simulink model "dynsim_edo_drag_gravity"  (R2020a)
settings: Solver=FixedStepAuto  StartTime=0.0  StopTime=10.0  FixedStep=0.001  RelTol=1e-3
libraries: robotlib x12, robotmaniplib x3
settings Model: Creator=bascetta  LastModifiedBy=alberto
settings OptimizationCC: EnhancedBackFolding=on  PassReuseOutputArgsAs=Individual arguments  ZeroExternalMemoryAtStartup=off  ZeroInternalMemoryAtStartup=off  MaxStackSize=64  OptimizeBlockOrder=speed  DifferentSizesBufferReuse=on  OptimizationCustomize=off  EfficientTunableParamExpr=on
settings DebuggingCC: ParameterTunabilityLossMsg=error
settings HardwareCC: ProdBitPerPointer=32  ProdBitPerSizeT=32  ProdBitPerPtrDiffT=32  ProdLargestAtomicFloat=None  ProdIntDivRoundTo=Undefined  ProdEndianess=Unspecified  ProdWordSize=32  ProdHWDeviceType=Generic->Unspecified (assume 32-bit Generic)
settings RTWCC: SystemTargetFile=ert.tlc  HardwareBoard=Robot Operating System (ROS)  TemplateMakefile=ert_default_tmf  GenerateReport=on  Toolchain=Catkin  IncludeHyperlinkInReport=on  LaunchReport=on  TargetLang=C++  GenerateTraceInfo=on  GenerateTraceReport=on  GenerateTraceReportSl=on  GenerateTraceReportSf=on  GenerateTraceReportEml=on
settings CodeAppCC: ForceParamTrailComments=on  IgnoreCustomStorageClasses=off  OperatorAnnotations=on  SimulinkDataObjDesc=on  SFDataObjDesc=on  InsertBlockDesc=on
settings ERTTargetCC: SupportContinuousTime=on  SupportVariableSizeSignals=on

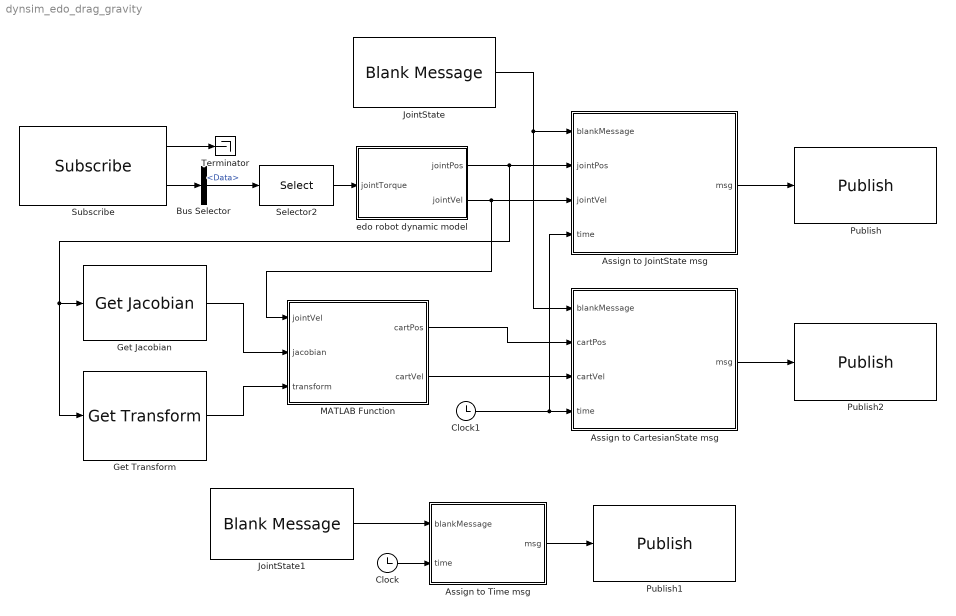
== system dynsim_edo_drag_gravity ==
  Assign to CartesianState msg : MATLAB Function  TreatAsAtomicUnit=on
  Assign to JointState msg : MATLAB Function  TreatAsAtomicUnit=on
  Assign to Time msg : MATLAB Function  TreatAsAtomicUnit=on
  Bus Selector : BusSelector  OutputSignals=Data
  Clock : Clock
  Clock1 : Clock
  Get Jacobian : robotmaniplib/Get Jacobian  RigidBodyTree=robot_edo  EndEffector=link_4  SimulateUsing=Interpreted execution
      settings: SourceProductBaseCode=RO
  Get Transform : robotmaniplib/Get Transform  RigidBodyTree=robot_edo  SourceBody=link_4  TargetBody=base_link  SimulateUsing=Interpreted execution
  JointState : robotlib/Blank Message  messageClass=Message  entityType=sensor_msgs/JointState  messageType=sensor_msgs/JointState  SampleTime=inf
  JointState1 : robotlib/Blank Message  messageClass=Message  entityType=rosgraph_msgs/Clock  messageType=rosgraph_msgs/Clock  SampleTime=inf
  MATLAB Function : MATLAB Function  TreatAsAtomicUnit=on
  Publish : robotlib/Publish  topicSource=Specify your own  topic=/joint_states  messageType=sensor_msgs/JointState  messageQueueLength=1
  Publish1 : robotlib/Publish  topicSource=Specify your own  topic=/clock  messageType=rosgraph_msgs/Clock  messageQueueLength=1
  Publish2 : robotlib/Publish  topicSource=Specify your own  topic=/cartesian_states  messageType=sensor_msgs/JointState  messageQueueLength=1
  Selector2 : Selector  IndexOptions=Starting index (dialog)  Indices=[2]  OutputSizes=3
  Subscribe : robotlib/Subscribe  topicSource=Specify your own  topic=/joint_torque  messageType=std_msgs/Float64MultiArray  sampleTime=-1  messageQueueLength=1
  Terminator : Terminator
  edo robot dynamic model : Subsystem
  wires:
  JointState1/1 -> Assign to Time msg/1(blankMessage)
  Assign to Time msg/1(msg) -> Publish1/1
  Subscribe/2 -> Bus Selector/1
  Subscribe/1 -> Terminator/1
  Selector2/1 -> edo robot dynamic model/1(jointTorque)
  Assign to JointState msg/1(msg) -> Publish/1
  edo robot dynamic model/2(jointVel) -> MATLAB Function/1(jointVel), Assign to JointState msg/3(jointVel)
  Bus Selector/1 -> Selector2/1  "<Data>"
  edo robot dynamic model/1(jointPos) -> Get Transform/1, Get Jacobian/1, Assign to JointState msg/2(jointPos)
  Clock/1 -> Assign to Time msg/2(time)
  Clock1/1 -> Assign to CartesianState msg/4(time), Assign to JointState msg/4(time)
  MATLAB Function/2(cartVel) -> Assign to CartesianState msg/3(cartVel)
  Assign to CartesianState msg/1(msg) -> Publish2/1
  MATLAB Function/1(cartPos) -> Assign to CartesianState msg/2(cartPos)
  JointState/1 -> Assign to CartesianState msg/1(blankMessage), Assign to JointState msg/1(blankMessage)
  Get Jacobian/1 -> MATLAB Function/2(jacobian)
  Get Transform/1 -> MATLAB Function/3(transform)

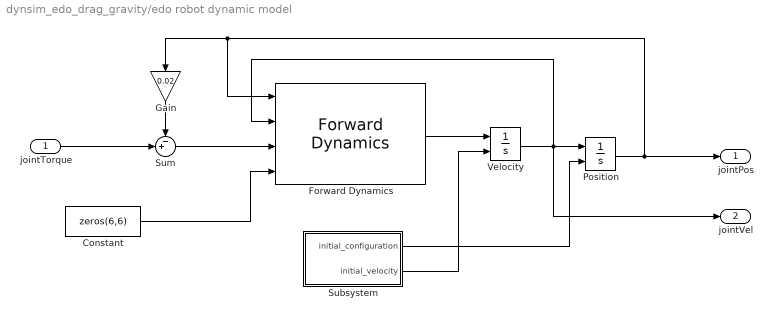
== system dynsim_edo_drag_gravity/edo robot dynamic model ==
  jointTorque : Inport
  Constant : Constant  Value=zeros(6,6)
  Forward Dynamics : robotmaniplib/Forward Dynamics  RigidBodyTree=robot_edo_nuove_inerzie  SimulateUsing=Interpreted execution
  Gain : Gain  Gain=0.02
  Position : Integrator  InitialConditionSource=external
  Subsystem : Subsystem
  Sum : Sum  Inputs=-+|
  Velocity : Integrator  InitialConditionSource=external
  jointPos : Outport
  jointVel : Outport  Port=2
  wires:
  Forward Dynamics/1 -> Velocity/1
  Position/1 -> Gain/1, Forward Dynamics/1, jointPos/1
  Constant/1 -> Forward Dynamics/4
  Velocity/1 -> Forward Dynamics/2, Position/1, jointVel/1
  Subsystem/2(initial_velocity) -> Velocity/2
  Subsystem/1(initial_configuration) -> Position/2
  jointTorque/1 -> Sum/2
  Sum/1 -> Forward Dynamics/3
  Gain/1 -> Sum/1

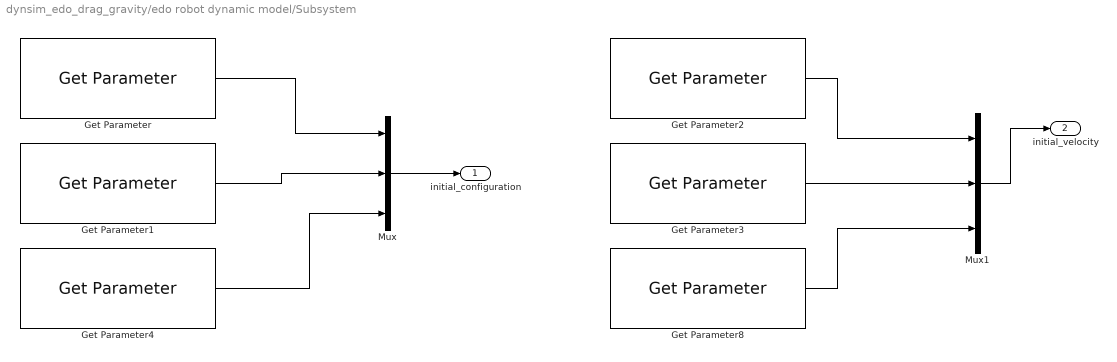
== system dynsim_edo_drag_gravity/edo robot dynamic model/Subsystem ==
  Get Parameter : robotlib/Get Parameter  ParameterSource=Specify your own  ParameterName=/dynsim_edo/q1_initial  ParameterType=double  ParameterMaxArrayLength=16  ParameterInitialValue=pi/4  SampleTime=-1  ShowErrorCodeOutput=off  ModelName=dynsim_edo_drag_gravity  BlockId=ParamGet_dynsim_edo_drag_gravity_112
      settings: SourceProductBaseCode=RR
  Get Parameter1 : robotlib/Get Parameter  ParameterSource=Specify your own  ParameterName=/dynsim_edo/q2_initial  ParameterType=double  ParameterMaxArrayLength=16  ParameterInitialValue=-pi/2  SampleTime=-1  ShowErrorCodeOutput=off  ModelName=dynsim_edo_drag_gravity  BlockId=ParamGet_dynsim_edo_drag_gravity_113
      settings: SourceProductBaseCode=RR
  Get Parameter2 : robotlib/Get Parameter  ParameterSource=Specify your own  ParameterName=/dynsim_edo/qv1_initial  ParameterType=double  ParameterMaxArrayLength=16  ParameterInitialValue=0  SampleTime=-1  ShowErrorCodeOutput=off  ModelName=dynsim_edo_drag_gravity  BlockId=ParamGet_dynsim_edo_drag_gravity_117
      settings: SourceProductBaseCode=RR
  Get Parameter3 : robotlib/Get Parameter  ParameterSource=Specify your own  ParameterName=/dynnsim_edo/qv2_initial  ParameterType=double  ParameterMaxArrayLength=16  ParameterInitialValue=0  SampleTime=-1  ShowErrorCodeOutput=off  ModelName=dynsim_edo_drag_gravity  BlockId=ParamGet_dynsim_edo_drag_gravity_118
      settings: SourceProductBaseCode=RR
  Get Parameter4 : robotlib/Get Parameter  ParameterSource=Specify your own  ParameterName=/dynsim_edo/q3_initial  ParameterType=double  ParameterMaxArrayLength=16  ParameterInitialValue=-pi/2  SampleTime=-1  ShowErrorCodeOutput=off  ModelName=dynsim_edo_drag_gravity  BlockId=ParamGet_dynsim_edo_drag_gravity_125
      settings: SourceProductBaseCode=RR
  Get Parameter8 : robotlib/Get Parameter  ParameterSource=Specify your own  ParameterName=/dynnsim_edo/qv3_initial  ParameterType=double  ParameterMaxArrayLength=16  ParameterInitialValue=0  SampleTime=-1  ShowErrorCodeOutput=off  ModelName=dynsim_edo_drag_gravity  BlockId=ParamGet_dynsim_edo_drag_gravity_133
      settings: SourceProductBaseCode=RR
  Mux : Mux  Inputs=3
  Mux1 : Mux  Inputs=3
  initial_configuration : Outport
  initial_velocity : Outport  Port=2
  wires:
  Mux/1 -> initial_configuration/1
  Get Parameter/1 -> Mux/1
  Get Parameter1/1 -> Mux/2
  Get Parameter3/1 -> Mux1/2
  Get Parameter2/1 -> Mux1/1
  Mux1/1 -> initial_velocity/1
  Get Parameter4/1 -> Mux/3
  Get Parameter8/1 -> Mux1/3

== matlab function dynsim_edo_drag_gravity/Assign to Time msg ==
  data: blankMessage input; msg output Bus: SL_Bus_dynsim_edo_drag_gravity_rosgraph_msgs_Clock; time input
function msg = assign_Time(blankMessage,time)
%#codegen

% Assign the output message to be the same with input blank message
msg = blankMessage;

% Convert and set time
msg.Clock_.Sec  = fix(time);
msg.Clock_.Nsec = fix((time-fix(time))*1e9);

== matlab function dynsim_edo_drag_gravity/Assign to JointState msg ==
  data: blankMessage input; msg output Bus: SL_Bus_dynsim_edo_drag_gravity_sensor_msgs_JointState; jointPos input; jointVel input; time input
function msg = assign_JointState(blankMessage,jointPos,jointVel,time)
%#codegen

% Assign the output message to be the same with input blank message
msg = blankMessage;

% Initialize time stamp
msg.Header.Stamp.Sec  = fix(time);
msg.Header.Stamp.Nsec = fix((time-fix(time))*1e9);

% Set the number of strings in the string array, and joint positions/velocities in the position/velocity array
numJoints = length(jointPos);
msg.Name_SL_Info.CurrentLength = uint32(numJoints);
msg.Position_SL_Info.CurrentLength = uint32(numJoints);
msg.Velocity_SL_Info.CurrentLength = uint32(numJoints);

% Set the individual components in the message arrays
strArrayToAssign = {'joint_1', 'joint_2', 'joint_3'};

for idx=1:numJoints
    str = strArrayToAssign{idx};
    strLength = length(str);
    msg.Name(idx).Data(1:strLength) = uint8(str);
    msg.Name(idx).Data_SL_Info.CurrentLength = uint32(strLength);

    msg.Position(idx) = jointPos(idx);
    msg.Velocity(idx) = jointVel(idx);
end

== matlab function dynsim_edo_drag_gravity/MATLAB Function ==
  data: jointVel input; jacobian input; cartPos output; transform input; cartVel output
function [cartPos,cartVel] = get_cartesian_values(jointVel,jacobian,transform)

cartVel = jacobian(3:6,:)*jointVel;

cartPos = transform(1:3,4);

== matlab function dynsim_edo_drag_gravity/Assign to CartesianState msg ==
  data: blankMessage input; msg output Bus: SL_Bus_dynsim_edo_drag_gravity_sensor_msgs_JointState; cartPos input; cartVel input; time input
function msg = assign_CartesianState(blankMessage,cartPos,cartVel,time)
%#codegen

% Assign the output message to be the same with input blank message
msg = blankMessage;

% Initialize time stamp
msg.Header.Stamp.Sec  = fix(time);
msg.Header.Stamp.Nsec = fix((time-fix(time))*1e9);

% Set the number of strings in the string array, and joint positions/velocities in the position/velocity array
numCoordinates = length(cartPos);
msg.Name_SL_Info.CurrentLength = uint32(numCoordinates);
msg.Position_SL_Info.CurrentLength = uint32(numCoordinates);
msg.Velocity_SL_Info.CurrentLength = uint32(numCoordinates);

% Set the individual components in the message arrays
strArrayToAssign = {'x_coord','y_coord','z_coord'};

for idx=1:numCoordinates
    str = strArrayToAssign{idx};
    strLength = length(str);
    msg.Name(idx).Data(1:strLength) = uint8(str);
    msg.Name(idx).Data_SL_Info.CurrentLength = uint32(strLength);

    msg.Position(idx) = cartPos(idx);
    msg.Velocity(idx) = cartVel(idx);
end
